simulink library "thc"  (R2021b)
settings: Solver=VariableStepAuto  StartTime=0.0  StopTime=10.0  RelTol=1e-3
undefined symbols (not defined in the file or in its folder): ATHC_APTCQA_X_C, ATHC_APTCQB_X_C, ATHC_dAy_X_C, ATHC_Qeq_X_kmh, ATHC_VbaseC_X_C, ATHC_VbaseC_Y_W, ATHC_VbaseD_X_C, ATHC_VbaseH_X_C, FALSE, KTHC_ACMaxMinT_sec, KTHC_aDeice_K, KTHC_AGSDefLv_K, KTHC_AGSLv1_K, KTHC_AGSLv2_K, KTHC_AGSLv3_K, KTHC_AGSLv4_K, KTHC_AGSLv5_K, KTHC_AirIntUpdateT_sec, KTHC_APTCOneZoneMax_W, KTHC_APTCPeriod_cnt, KTHC_APTCPWMEN_flg, KTHC_APTCQMaxC_W, KTHC_APTCQminC_W, KTHC_APTCQminD_W, KTHC_APTCQminRe1_W, KTHC_APTCQminRe_W, KTHC_APTCQoffT_cnt, KTHC_APTCQonT_cnt, KTHC_APTCRiLeMaxDff_W, KTHC_APTCRiLeMinDff_W, KTHC_BatInTempDef_C, KTHC_bDeice_K, KTHC_CompMaxDeice_rpm, KTHC_CompMinDeice_rpm, KTHC_CompSotxvOp_K, KTHC_CompSotxvOpLow_rpm, KTHC_CompSpdmax_rpm, KTHC_CompSpdmaxBC1_rpm, KTHC_CompSpdmaxBC_rpm, KTHC_CompSpdmid1_rpm, KTHC_CompSpdmid2_rpm, KTHC_CompSpdmid3_rpm, KTHC_CompSpdmid_rpm, KTHC_CompSpdmin_rpm, KTHC_DAPTCQ1_W, KTHC_DAPTCQ2_W, KTHC_DAPTCQ3_W, KTHC_DcChSetTemp_C, KTHC_DehumidityEN_flg, KTHC_DeiceCycTime_K, KTHC_DriveLevelWPTCBAH1_W, KTHC_DriveLevelWPTCBAH2_W, KTHC_DriveLevelWPTCBAH3_W, KTHC_DriveLevelWPTCBAH4_W, KTHC_DriveT1MinBAH_C, KTHC_DriveT2MaxBAH_C, KTHC_DriveT2MinBAH_C, KTHC_DriveT3MaxBAH_C, KTHC_DriveT3MinBAH_C, KTHC_DriveT4MaxBAH_C ... (+372)
libraries: simulink x140
(part 2 of 10)

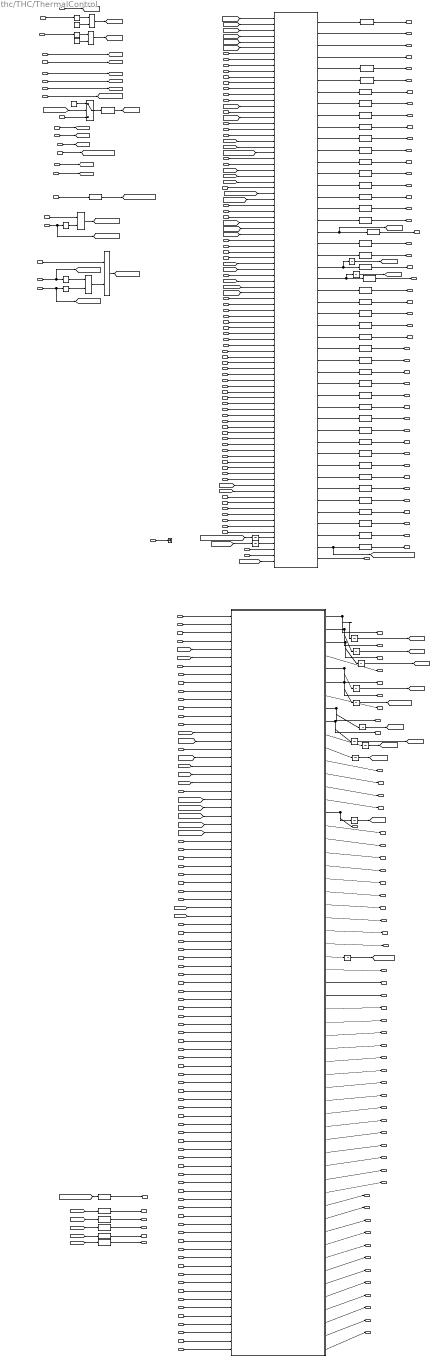
== system thc/THC/ThermalControl ==
  note: Ver Infomation
      | THCM Model V86test2A
      | ACHMI Model V27A
  VPMM_PwrSta_enum : Inport
  VTQD_ShiftGearPosn_enum : Inport  Port=2
  VSCP_AGSCloseSta_flg : Inport  Port=3
  VINP_VehSpeed_kph : Inport  Port=4
  VINP_HVBMTempMax_C : Inport  Port=5
  VINP_HVBMTempMin_C : Inport  Port=6
  VINP_OBCTemp_C : Inport  Port=7
  VINP_DCDCTemp_C : Inport  Port=8
  VINP_RrTMTemp_C : Inport  Port=9
  VINP_RrMCUTemp_C : Inport  Port=10
  VINP_FrTMTemp_C : Inport  Port=11
  VINP_FrMCUTemp_C : Inport  Port=12
  VINP_ChrgPlugSta_enum : Inport  Port=13
  VINP_FrLLCTemp_C : Inport  Port=14
  VINP_RrLLCTemp_C : Inport  Port=15
  VINP_HVBIsoImpedenceN_Mohm : Inport  Port=16
  VINP_HVBIsoImpedenceP_Mohm : Inport  Port=17
  VINP_HVBHVILErr_flg : Inport  Port=18
  VINP_HVBattSOC_pct : Inport  Port=19
  VINP_PTHighTact_C : Inport  Port=20
  VINP_COMP_StatorSpd_RPM : Inport  Port=21
  VINP_CompProEN_flg : Inport  Port=22
  VINP_PTLowP1_kPa : Inport  Port=23
  VINP_PTLowT1_C : Inport  Port=24
  VINP_PTLowP2_kPa : Inport  Port=25
  VINP_PTLowT2_C : Inport  Port=26
  VINP_PTHighP_kPa : Inport  Port=27
  VINP_Tamb_C : Inport  Port=28
  VINP_BatInTemp_C : Inport  Port=29
  VINP_BatOutTemp_C : Inport  Port=30
  VINP_MotorInTemp_C : Inport  Port=31
  VINP_MotorOutTemp_C : Inport  Port=32
  VINP_Tincar_C : Inport  Port=33
  VINP_SolarL_W : Inport  Port=34
  VINP_SolarR_W : Inport  Port=35
  VINP_Tevap_C : Inport  Port=36
  VINP_TFaceL_C : Inport  Port=37
  VINP_TFaceR_C : Inport  Port=38
  VINP_TFootL_C : Inport  Port=39
  VINP_TFootR_C : Inport  Port=40
  VINP_TFootRr_C : Inport  Port=41
  VINP_TFaceRr_C : Inport  Port=42
  VINP_EACProtectEnable_enum : Inport  Port=43
  Tamb_Err : Inport  Port=44
  SolarL_Err : Inport  Port=45
  SolarR_Err : Inport  Port=46
  Tevap_Err : Inport  Port=47
  T_Face_L_Err : Inport  Port=48
  T_Face_R_Err : Inport  Port=49
  T_Foot_L_Err : Inport  Port=50
  T_Foot_R_Err : Inport  Port=51
  T_Face_Rr_Err : Inport  Port=52
  T_Foot_Rr_Err : Inport  Port=53
  Tincar_Err : Inport  Port=54
  Bat_In_Temp_Err : Inport  Port=55
  Motor_In_Temp_Err : Inport  Port=56
  Motor_Out_Temp_Err : Inport  Port=57
  Fan_Err : Inport  Port=58
  AGS_Err : Inport  Port=59
  EWP3_Err : Inport  Port=60
  PT_High_P_Err : Inport  Port=61
  PT_High_Tact_Err : Inport  Port=62
  SOV1_Err : Inport  Port=63
  SOV2_Err : Inport  Port=64
  SOV3_Err : Inport  Port=65
  EXV1_Err : Inport  Port=66
  EXV2_Err : Inport  Port=67
  Comp_Err : Inport  Port=68
  Blower_Err : Inport  Port=69
  PT_Low_P1_Err : Inport  Port=70
  PT_Low_T1_Err : Inport  Port=71
  PT_Low_P2_Err : Inport  Port=72
  PT_Low_T2_Err : Inport  Port=73
  SOTXV_Err : Inport  Port=74
  VINP_FrntPTCRearLeActHeatPwr_W : Inport  Port=75
  VINP_FrntPTCRearRiActHeatPwr_W : Inport  Port=76
  VINP_FrntPTCRiActHeatPwr_W : Inport  Port=77
  VINP_ZFRTHCDrEVentActYSta_enum : Inport  Port=78
  VINP_ZFRTHCCLEVentActYSta_enum : Inport  Port=79
  VINP_ZFRTHCPsEVentActYSta_enum : Inport  Port=80
  VINP_ZFRTHCCREVentActYSta_enum : Inport  Port=81
  VINP_FGSAirIntSta_enum : Inport  Port=82
  VINP_FGSMotorInitSta_enum : Inport  Port=83
  VINP_OFFACMODE_enum : Inport  Port=84
  VINP_FCPFrEvtBtnACMaxReq_flg : Inport  Port=85
  VINP_FCPFrEvtBtnACReq_flg : Inport  Port=86
  VINP_FCPFrEvtBtnAutoReq_flg : Inport  Port=87
  VINP_FCPFrEvtBtnSyncReq_flg : Inport  Port=88
  VINP_sigAirIntenZon1Req_enum : Inport  Port=89
  VINP_sigRecircReq_flg : Inport  Port=90
  VINP_sigFaceReq_flg : Inport  Port=91
  VINP_sigFootReq_flg : Inport  Port=92
  VINP_sigFrostReq_flg : Inport  Port=93
  VINP_sigSetTempZon1Req_C : Inport  Port=94
  VINP_CANMsgValidIVI2_flg : Inport  Port=95
  VINP_sigSetTempZon2Req_C : Inport  Port=96
  VINP_SmartEcoModeSW_flg : Inport  Port=97
  VINP_HMIACBtnCmd_flg : Inport  Port=98
  VINP_HMIACAutoBtnCmd_flg : Inport  Port=99
  VINP_HMIACRecycleBtnCmd_flg : Inport  Port=100
  VINP_HMIACFrDefogBtnCmd_flg : Inport  Port=101
  VINP_HMIZ1SetTPCmd_flg : Inport  Port=102
  VINP_HMIZ1SetTMCmd_flg : Inport  Port=103
  VINP_HMIZ2SetTPCmd_flg : Inport  Port=104
  VINP_HMIZ2SetTMCmd_flg : Inport  Port=105
  VINP_HMIACWindDirPCmd_flg : Inport  Port=106
  VINP_HMIACWindDirMCmd_flg : Inport  Port=107
  VINP_HMIACAirIntPCmd_flg : Inport  Port=108
  VINP_HMIACAirIntDirMCmd_flg : Inport  Port=109
  VINP_IVIAirIntZ3Cmd_enum : Inport  Port=110
  VINP_IVIDrBlowerModeSta_enum : Inport  Port=111
  VINP_IVIPsBlowerModeSta_enum : Inport  Port=112
  VINP_IVIDrBlowerZSta_enum : Inport  Port=113
  VINP_IVICLBlowerZSta_enum : Inport  Port=114
  VINP_IVIPsBlowerZSta_enum : Inport  Port=115
  VINP_IVICRBlowerZSta_enum : Inport  Port=116
  VINP_IVIDrBlowerYSta_enum : Inport  Port=117
  VINP_IVICLBlowerYSta_enum : Inport  Port=118
  VINP_IVIPsBlowerYSta_enum : Inport  Port=119
  VINP_IVICRBlowerYSta_enum : Inport  Port=120
  VINP_IVIsigScreenReq_Sta : Inport  Port=121
  VINP_IVIFGSAirIntCmd_enum : Inport  Port=122
  VINP_IVIFGSChCmd_enum : Inport  Port=123
  VINP_IVIIONSWCmd_flg : Inport  Port=124
  VINP_IVIWPTCSWSta_flg : Inport  Port=125
  VINP_IVIZon1WindDirSWReqSta_flg : Inport  Port=126
  ECOSW : Inport  Port=127
  EEP_ACModeMem : Inport  Port=128
  EEP_Face : Inport  Port=129
  EEP_Foot : Inport  Port=130
  EEP_Frost : Inport  Port=131
  EEP_FaceM : Inport  Port=132
  EEP_FootM : Inport  Port=133
  EEP_CCUSyncSts : Inport  Port=134
  EEP_ACForceOFF : Inport  Port=135
  EEP_sigRecircSt : Inport  Port=136
  EEP_RecAutoFlg : Inport  Port=137
  EEP_AirIntenZone1iM : Inport  Port=138
  EEP_fdefog : Inport  Port=139
  EEP_sigSetTempZon1St : Inport  Port=140
  EEP_sigSetTempZon2StM : Inport  Port=141
  EEP_FDCTHCAirIntZ3Sta : Inport  Port=142
  VINP_FDCTHCPsEVentModeStaM_enum : Inport  Port=143
  VINP_FDCTHCDrEVentModeStaM_enum : Inport  Port=144
  VINP_FDCTHCDrEVentZStaM_enum : Inport  Port=145
  VINP_FDCTHCCLEVentZStaM_enum : Inport  Port=146
  VINP_FDCTHCPsEVentZStaM_enum : Inport  Port=147
  VINP_FDCTHCCREVentZStaM_enum : Inport  Port=148
  EEP_DrVentENM : Inport  Port=149
  VINP_FDCTHCDrEVentYStaM_enum : Inport  Port=150
  EEP_CLVentENM : Inport  Port=151
  VINP_FDCTHCCLEVentYStaM_enum : Inport  Port=152
  EEP_PsVentENM : Inport  Port=153
  VINP_FDCTHCPsEVentYStaM_enum : Inport  Port=154
  EEP_CRVentENM : Inport  Port=155
  VINP_FDCTHCCREVentYStaM_enum : Inport  Port=156
  FGSAirIntStaM : Inport  Port=157
  FGSChStaM : Inport  Port=158
  "IONSWStaM " : Inport  Port=159
  APTCFailDTC : Inport  Port=160
  VINP_RemoteACTemp_C : Inport  Port=161
  VINP_RemoteAutoReq_flg : Inport  Port=162
  AC1 : Subsystem
  Abs : Abs
  Abs1 : Abs
  Constant : Constant
  Constant1 : Constant
  Constant2 : Constant  Value=2
  Data Type Conversion{,1..47,50} (49 alike) : DataTypeConversion
  Data Type Conversion48 : DataTypeConversion  OutDataTypeStr=uint8
  Data Type Conversion49 : DataTypeConversion  OutDataTypeStr=uint16
  Logical Operator : Logic  Operator=OR  AllPortsSameDT=off  OutDataTypeStr=boolean
  Logical Operator1 : Logic  Operator=OR  AllPortsSameDT=off  OutDataTypeStr=boolean
  Logical Operator2 : Logic  AllPortsSameDT=off  OutDataTypeStr=boolean
  Logical Operator3 : Logic  Operator=NOT  AllPortsSameDT=off  OutDataTypeStr=boolean
  Logical Operator4 : Logic  Operator=NOT  AllPortsSameDT=off  OutDataTypeStr=boolean
  Logical Operator5 : Logic  Operator=NOT  AllPortsSameDT=off  OutDataTypeStr=boolean
  Max : MinMax  Function=max  Inputs=2
  Max1 : MinMax  Function=max  Inputs=2
  Switch : Switch  Criteria=u2 > Threshold
  THCM_Conctrl : Subsystem
  Terminator : Terminator
  Unit Delay{,1..14} (15 alike) : UnitDelay  SampleTime=-1  HasFrameUpgradeWarning=on
  VTHC_FDCompCmd_rpm : Outport
  VTHC_FDSOV1Cmd_flg : Outport  Port=2
  VTHC_FDSOV2Cmd_flg : Outport  Port=3
  VTHC_FDSOV3Cmd_flg : Outport  Port=4
  VTHC_FDEXV1Cmd_step : Outport  Port=5
  VTHC_FDEXV2Cmd_step : Outport  Port=6
  VTHC_FDSOTXVCmd_flg : Outport  Port=7
  VTHC_FDFWVCmd_flg : Outport  Port=8
  VTHC_FDTWVCmd_pct : Outport  Port=9
  VTHC_FDFrWPTCHeatPwrCmd_W : Outport  Port=10
  VTHC_CoolgFanActDuty_pct : Outport  Port=11
  VTHC_FDAGSCmd_enum : Outport  Port=12
  VTHC_FDEWP1Cmd_enum : Outport  Port=13
  VTHC_FDEWP2Cmd_enum : Outport  Port=14
  VTHC_FDEWP3Cmd_enum : Outport  Port=15
  VTHC_FDFrLeAPTCHeatPwrCmd_W : Outport  Port=16
  VTHC_FDFrRiAPTCHeatPwrCmd_W : Outport  Port=17
  VTHC_FDRrAPTCHeatPwrCmd_W : Outport  Port=18
  VTHC_FDBlowerCmd_pct : Outport  Port=19
  VTHC_BatteryMode_enum : Outport  Port=20
  VTHC_EDriveMode_enum : Outport  Port=21
  VTHC_CabinMode_enum : Outport  Port=22
  VTHC_CCUACLampSts_flg : Outport  Port=23
  VTHC_CCUAutoLampSts_flg : Outport  Port=24
  VTHC_CCUACMaxLampSts_flg : Outport  Port=25
  VTHC_CCUSyncLampSts_flg : Outport  Port=26
  VTHC_sigAirIntenZon1St_enum : Outport  Port=27
  VTHC_sigWindDirZon1St_enum : Outport  Port=28
  VTHC_sigRecircSt_flg : Outport  Port=29
  VTHC_sigSetTempZon1St_C : Outport  Port=30
  VTHC_sigSetTempZon2St_C : Outport  Port=31
  VTHC_sigClntTHvBattOut_C : Outport  Port=32
  VTHC_sigCbnSolarLeft_W : Outport  Port=33
  VTHC_sigClntTHvBattIn_C : Outport  Port=34
  VTHC_sigCbnSolarRight_W : Outport  Port=35
  VTHC_sigAmbAirT_C : Outport  Port=36
  VTHC_sigCbnAirT_C : Outport  Port=37
  VTHC_ACSubMode_enum : Outport  Port=38
  VTHC_FDRecyAutoCmd_enum : Outport  Port=39
  VTHC_CompP_K : Outport  Port=40
  VTHC_CompI_K : Outport  Port=41
  VTHC_CompU_K : Outport  Port=42
  VTHC_CompDeltaU_K : Outport  Port=43
  VTHC_Compe_K : Outport  Port=44
  VTHC_Blowere_K : Outport  Port=45
  VTHC_BlowerP_K : Outport  Port=46
  VTHC_BlowerU_K : Outport  Port=47
  VTHC_Vbase_pct : Outport  Port=48
  VTHC_BlowerI_K : Outport  Port=49
  VTHC_EXV2P_K : Outport  Port=50
  VTHC_EXV2I_K : Outport  Port=51
  VTHC_EXV2U_K : Outport  Port=52
  VTHC_EXV2e_K : Outport  Port=53
  VTHC_APTCP_K : Outport  Port=54
  VTHC_APTCI_K : Outport  Port=55
  VTHC_APTCU_K : Outport  Port=56
  VTHC_APTCe_K : Outport  Port=57
  VTHC_EXV1P_K : Outport  Port=58
  VTHC_EXV1I_K : Outport  Port=59
  VTHC_EXV1U_K : Outport  Port=60
  VTHC_EXV1e_K : Outport  Port=61
  VTHC_ACModeMem_enum : Outport  Port=62
  VTHC_Face_flg : Outport  Port=63
  VTHC_Foot_flg : Outport  Port=64
  VTHC_Frost_flg : Outport  Port=65
  VTHC_FaceM_flg : Outport  Port=66
  VTHC_FootM_flg : Outport  Port=67
  VTHC_CCUSyncSts_flg : Outport  Port=68
  VTHC_ACForceOFF_flg : Outport  Port=69
  VTHC_RecAutoFlg_flg : Outport  Port=70
  VTHC_AirIntenZone1M_enum : Outport  Port=71
  VTHC_fdefog_flg : Outport  Port=72
  VTHC_sigSetTempZon2StM_C : Outport  Port=73
  VTHC_sigDfrstSt_flg : Outport  Port=74
  VTHC_FDCTHCAirIntZ3Sta_enum : Outport  Port=75
  VTHC_FDCTHCDrEVentModeSta_enum : Outport  Port=76
  VTHC_FDCTHCPsEVentModeSta_enum : Outport  Port=77
  VTHC_FDCTHCDrEVentZSta_enum : Outport  Port=78
  VTHC_FDCTHCCLEVentZSta_enum : Outport  Port=79
  VTHC_FDCTHCPsEVentZSta_enum : Outport  Port=80
  VTHC_FDCTHCCREVentZSta_enum : Outport  Port=81
  VTHC_FDCTHCDrEVentYSta_enum : Outport  Port=82
  VTHC_FDCTHCDrVentENSta_flg : Outport  Port=83
  VTHC_FDCTHCCLEVentYSta_enum : Outport  Port=84
  VTHC_FDCTHCCLVentENSta_flg : Outport  Port=85
  VTHC_FDCTHCPsEVentYSta_enum : Outport  Port=86
  VTHC_FDCTHCPsVentENSta_flg : Outport  Port=87
  VTHC_FDCTHCCREVentYSta_enum : Outport  Port=88
  VTHC_FDCTHCCRVentENSta_flg : Outport  Port=89
  VTHC_FDCTHCMAPTCForceOFFSta_flg : Outport  Port=90
  VTHC_DrVentEN_flg : Outport  Port=91
  VTHC_CLVentEN_flg : Outport  Port=92
  VTHC_PsVentEN_flg : Outport  Port=93
  VTHC_CRVentEN_flg : Outport  Port=94
  VTHC_Z1TUP_flg : Outport  Port=95
  VTHC_Z1TDN_flg : Outport  Port=96
  VTHC_Z2TUP_flg : Outport  Port=97
  VTHC_Z2TDN_flg : Outport  Port=98
  VTHC_FDCFGSAirIntSta_enum : Outport  Port=99
  VTHC_FDCFGSChSta_enum : Outport  Port=100
  VTHC_FDCFGSAirIntCmd_enum : Outport  Port=101
  VTHC_FDCFGSFuncSta_flg : Outport  Port=102
  VTHC_FDCFGSChCmd_enum : Outport  Port=103
  VTHC_FDCFGSIONSWSta_flg : Outport  Port=104
  VTHC_FDCFGSIONCmd_flg : Outport  Port=105
  VTHC_FDCFGSLearnCmd_enum : Outport  Port=106
  VTHC_FDCTHCMPreWPTCHeatSta_enum : Outport  Port=107
  wires:
  AC1/9(VTHC_sigSetTempZon2St_C) -> Unit Delay9/1, VTHC_sigSetTempZon2St_C/1
  AC1/2(VTHC_CCUAutoLampSts_flg) -> Unit Delay2/1, VTHC_CCUAutoLampSts_flg/1
  AC1/6(VTHC_sigWindDirZon1St_enum) -> Unit Delay14/1, VTHC_sigWindDirZon1St_enum/1
  Unit Delay3/1 -> [ACMAX]
  AC1/4(VTHC_CCUSyncLampSts_flg) -> VTHC_CCUSyncLampSts_flg/1
  AC1/1(VTHC_CCUACLampSts_flg) -> Unit Delay1/1, VTHC_CCUACLampSts_flg/1
  AC1/5(VTHC_sigAirIntenZon1St_enum) -> Unit Delay4/1, VTHC_sigAirIntenZon1St_enum/1
  AC1/8(VTHC_sigSetTempZon1St_C) -> Unit Delay5/1, VTHC_sigSetTempZon1St_C/1
  THCM_Conctrl/19(FD_Blower_Cmd) -> Data Type Conversion/1, [FD_Blower_Cmd]
  Unit Delay5/1 -> [sigSetTempZon1St]
  AC1/7(VTHC_sigRecircSt_flg) -> VTHC_sigRecircSt_flg/1
  AC1/3(VTHC_CCUACMaxLampSts_flg) -> Unit Delay3/1, VTHC_CCUACMaxLampSts_flg/1
  VPMM_PwrSta_enum/1 -> [PwrSta]
  THCM_Conctrl/13(FD_EWP1_Cmd) -> Data Type Conversion3/1
  THCM_Conctrl/11(CoolgFanActDuty) -> Data Type Conversion1/1
  THCM_Conctrl/18(FD_RrAPTCHeatPwr_Cmd) -> Data Type Conversion8/1
  THCM_Conctrl/21(EDriveMode) -> Data Type Conversion22/1
  THCM_Conctrl/20(BatteryMode) -> Data Type Conversion21/1
  THCM_Conctrl/16(FD_FrLeAPTCHeatPwr_Cmd) -> Data Type Conversion6/1
  VINP_Tincar_C/1 -> [Tincar]
  THCM_Conctrl/9(FD_TWV_Cmd) -> Data Type Conversion19/1
  THCM_Conctrl/4(FD_SOV3_Cmd) -> VTHC_FDSOV3Cmd_flg/1
  VINP_SolarR_W/1 -> [SolarR]
  THCM_Conctrl/15(FD_EWP3_Cmd) -> Data Type Conversion5/1
  THCM_Conctrl/2(FD_SOV1_Cmd) -> VTHC_FDSOV1Cmd_flg/1
  Unit Delay2/1 -> [ACAUTO]
  THCM_Conctrl/7(FD_SOTXV_Cmd) -> Data Type Conversion46/1
  THCM_Conctrl/14(FD_EWP2_Cmd) -> Data Type Conversion4/1
  THCM_Conctrl/3(FD_SOV2_Cmd) -> VTHC_FDSOV2Cmd_flg/1
  THCM_Conctrl/6(FD_EXV2_Cmd) -> Data Type Conversion17/1
  VINP_Tamb_C/1 -> [Tamb]
  THCM_Conctrl/8(FD_FWV_Cmd) -> Data Type Conversion18/1
  VINP_BatInTemp_C/1 -> [BatInTemp]
  Unit Delay1/1 -> [AC]
  THCM_Conctrl/17(FD_FrRiAPTCHeatPwr_Cmd) -> Data Type Conversion7/1
  VINP_SolarL_W/1 -> [SolarL]
  THCM_Conctrl/12(FD_AGS_Cmd) -> Data Type Conversion2/1
  VINP_TFootL_C/1 -> [TFootL]
  Unit Delay4/1 -> [sigAirIntenZon1St]
  THCM_Conctrl/10(FD_FrWPTCHeatPwr_Cmd) -> Data Type Conversion20/1
  THCM_Conctrl/22(CabinMode) -> Unit Delay11/1, Data Type Conversion23/1
  [SolarL] -> Data Type Conversion41/1  "VTHC_sigCbnSolarLeft_W"
  [SolarR] -> Data Type Conversion43/1  "VTHC_sigCbnSolarRight_W"
  [BatInTemp] -> Data Type Conversion42/1  "VTHC_sigClntTHvBattIn_C"
  [Tamb] -> Data Type Conversion44/1  "VTHC_sigAmbAirT_C"
  [Tincar] -> Data Type Conversion45/1  "VTHC_sigCbnAirT_C"
  VINP_PTLowP2_kPa/1 -> Abs/1
  Abs/1 -> Max/1
  Constant/1 -> Max/2
  Constant1/1 -> Max1/2
  Abs1/1 -> Max1/1
  VINP_PTLowP1_kPa/1 -> Abs1/1
  VINP_TFootR_C/1 -> [TFootR]
  VINP_TFootRr_C/1 -> [TFootRr]
  VINP_CompProEN_flg/1 -> [VINP_CompProEN_flg]
  THCM_Conctrl/23(ACSubMode) -> Data Type Conversion28/1, Unit Delay/1
  THCM_Conctrl/24(VTHC_CompP_K) -> Data Type Conversion29/1
  THCM_Conctrl/25(VTHC_CompI_K) -> Data Type Conversion35/1
  THCM_Conctrl/26(VTHC_CompU_K) -> Data Type Conversion36/1
  THCM_Conctrl/27(VTHC_CompDeltaU_K) -> Data Type Conversion34/1
  THCM_Conctrl/28(VTHC_Compe_K) -> Data Type Conversion33/1
  THCM_Conctrl/29(VTHC_Blowere_K) -> Data Type Conversion32/1
  THCM_Conctrl/30(VTHC_BlowerP_K) -> Data Type Conversion31/1
  THCM_Conctrl/31(VTHC_BlowerU_K) -> Data Type Conversion30/1
  THCM_Conctrl/32(VTHC_Vbase_pct) -> Data Type Conversion37/1
  THCM_Conctrl/33(VTHC_BlowerI_K) -> Data Type Conversion38/1
  THCM_Conctrl/34(VTHC_EXV2P_K) -> Data Type Conversion24/1
  THCM_Conctrl/35(VTHC_EXV2I_K) -> Data Type Conversion25/1
  THCM_Conctrl/36(VTHC_EXV2U_K) -> Data Type Conversion26/1
  THCM_Conctrl/37(VTHC_EXV2e_K) -> Data Type Conversion27/1
  THCM_Conctrl/39(VTHC_APTCI_K) -> Data Type Conversion16/1
  THCM_Conctrl/40(VTHC_APTCU_K) -> Data Type Conversion15/1
  THCM_Conctrl/41(VTHC_APTCe_K) -> Data Type Conversion14/1
  THCM_Conctrl/42(VTHC_EXV1P_K) -> Data Type Conversion11/1
  THCM_Conctrl/43(VTHC_EXV1I_K) -> Data Type Conversion12/1
  THCM_Conctrl/44(VTHC_EXV1U_K) -> Data Type Conversion13/1
  THCM_Conctrl/45(VTHC_EXV1e_K) -> Data Type Conversion9/1
  THCM_Conctrl/5(FD_EXV1_Cmd) -> Data Type Conversion10/1
  Data Type Conversion1/1 -> VTHC_CoolgFanActDuty_pct/1  "CoolgFanActDuty"
  Data Type Conversion2/1 -> VTHC_FDAGSCmd_enum/1  "FD_AGS_Cmd"
  Data Type Conversion3/1 -> VTHC_FDEWP1Cmd_enum/1  "FD_EWP1_Cmd"
  Data Type Conversion4/1 -> VTHC_FDEWP2Cmd_enum/1  "FD_EWP2_Cmd"
  Data Type Conversion5/1 -> VTHC_FDEWP3Cmd_enum/1  "FD_EWP3_Cmd"
  Data Type Conversion6/1 -> VTHC_FDFrLeAPTCHeatPwrCmd_W/1  "FD_FrLeAPTCHeatPwr_Cmd"
  Data Type Conversion8/1 -> VTHC_FDRrAPTCHeatPwrCmd_W/1  "FD_RrAPTCHeatPwr_Cmd"
  Data Type Conversion7/1 -> VTHC_FDFrRiAPTCHeatPwrCmd_W/1  "FD_FrRiAPTCHeatPwr_Cmd"
  Data Type Conversion9/1 -> VTHC_EXV1e_K/1  "VTHC_EXV1e_K"
  Data Type Conversion10/1 -> VTHC_FDEXV1Cmd_step/1  "FD_EXV1_Cmd"
  Data Type Conversion11/1 -> VTHC_EXV1P_K/1  "VTHC_EXV1P_K"
  Data Type Conversion12/1 -> VTHC_EXV1I_K/1  "VTHC_EXV1I_K"
  Data Type Conversion13/1 -> VTHC_EXV1U_K/1  "VTHC_EXV1U_K"
  Data Type Conversion14/1 -> VTHC_APTCe_K/1  "VTHC_APTCe_K"
  Data Type Conversion15/1 -> VTHC_APTCU_K/1  "VTHC_APTCU_K"
  Data Type Conversion16/1 -> VTHC_APTCI_K/1  "VTHC_APTCI_K"
  THCM_Conctrl/38(VTHC_APTCP_K) -> Data Type Conversion39/1
  Data Type Conversion17/1 -> VTHC_FDEXV2Cmd_step/1  "FD_EXV2_Cmd"
  Data Type Conversion18/1 -> VTHC_FDFWVCmd_flg/1  "FD_FWV_Cmd"
  Data Type Conversion19/1 -> VTHC_FDTWVCmd_pct/1  "FD_TWV_Cmd"
  Data Type Conversion20/1 -> VTHC_FDFrWPTCHeatPwrCmd_W/1  "FD_FrWPTCHeatPwr_Cmd"
  Data Type Conversion21/1 -> VTHC_BatteryMode_enum/1  "BatteryMode"
  Data Type Conversion22/1 -> VTHC_EDriveMode_enum/1  "EDriveMode"
  Data Type Conversion23/1 -> VTHC_CabinMode_enum/1  "CabinMode"
  Data Type Conversion24/1 -> VTHC_EXV2P_K/1  "VTHC_EXV2P_K"
  Data Type Conversion25/1 -> VTHC_EXV2I_K/1  "VTHC_EXV2I_K"
  Data Type Conversion26/1 -> VTHC_EXV2U_K/1  "VTHC_EXV2U_K"
  Data Type Conversion27/1 -> VTHC_EXV2e_K/1  "VTHC_EXV2e_K"
  Data Type Conversion28/1 -> VTHC_ACSubMode_enum/1  "ACSubMode"
  Data Type Conversion29/1 -> VTHC_CompP_K/1  "VTHC_CompP_K"
  Data Type Conversion30/1 -> VTHC_BlowerU_K/1  "VTHC_BlowerU_K"
  Data Type Conversion31/1 -> VTHC_BlowerP_K/1  "VTHC_BlowerP_K"
  Data Type Conversion32/1 -> VTHC_Blowere_K/1  "VTHC_Blowere_K"
  Data Type Conversion33/1 -> VTHC_Compe_K/1  "VTHC_Compe_K"
  Data Type Conversion34/1 -> VTHC_CompDeltaU_K/1  "VTHC_CompDeltaU_K"
  Data Type Conversion35/1 -> VTHC_CompI_K/1  "VTHC_CompI_K"
  Data Type Conversion36/1 -> VTHC_CompU_K/1  "VTHC_CompU_K"
  Data Type Conversion37/1 -> VTHC_Vbase_pct/1  "VTHC_Vbase_pct"
  Data Type Conversion38/1 -> VTHC_BlowerI_K/1  "VTHC_BlowerI_K"
  Data Type Conversion39/1 -> VTHC_APTCP_K/1  "VTHC_APTCP_K"
  Data Type Conversion40/1 -> VTHC_sigClntTHvBattOut_C/1  "VINP_BatOutTemp_C"
  Data Type Conversion41/1 -> VTHC_sigCbnSolarLeft_W/1  "SolarL"
  Data Type Conversion42/1 -> VTHC_sigClntTHvBattIn_C/1  "BatInTemp"
  Data Type Conversion43/1 -> VTHC_sigCbnSolarRight_W/1  "SolarR"
  Data Type Conversion44/1 -> VTHC_sigAmbAirT_C/1  "Tamb"
  Data Type Conversion45/1 -> VTHC_sigCbnAirT_C/1  "Tincar"
  AC1/10(WaterFillReq) -> Unit Delay7/1
  AC1/16(Frost) -> Unit Delay8/1, VTHC_Frost_flg/1
  Unit Delay8/1 -> [DfrstReq]
  Unit Delay7/1 -> [WaterFillReq]
  Unit Delay9/1 -> [sigSetTempZon2St]
  Data Type Conversion/1 -> VTHC_FDBlowerCmd_pct/1
  Data Type Conversion46/1 -> VTHC_FDSOTXVCmd_flg/1
  VINP_BatOutTemp_C/1 -> [VINP_BatOutTemp_C]
  [VINP_BatOutTemp_C] -> Data Type Conversion40/1
  AC1/11(PET) -> Unit Delay10/1
  Unit Delay10/1 -> [PET]
  THCM_Conctrl/1(FD_Comp_Cmd) -> Data Type Conversion47/1
  Data Type Conversion47/1 -> VTHC_FDCompCmd_rpm/1  "VTHC_FDCompCmd_rpm"
  Unit Delay11/1 -> [CabinMode]
  AC1/12(FD_RecyAuto_Cmd) -> VTHC_FDRecyAutoCmd_enum/1
  [VINP_CompProEN_flg] -> Switch/2
  Switch/1 -> Data Type Conversion48/1
  Constant2/1 -> Switch/1
  VINP_EACProtectEnable_enum/1 -> Switch/3
  Max1/1 -> [PTLowP1]
  Max/1 -> [PTLowP2]
  [PwrSta] -> THCM_Conctrl/1(PwrSta)
  [AC] -> THCM_Conctrl/2(AC)
  [ACMAX] -> THCM_Conctrl/3(ACMax)
  [ACAUTO] -> THCM_Conctrl/4(ACAuto)
  [sigSetTempZon1St] -> THCM_Conctrl/5(sigSetTempZon1St)
  [sigAirIntenZon1St] -> THCM_Conctrl/6(sigAirIntenZon1St)
  VINP_VehSpeed_kph/1 -> THCM_Conctrl/7(VehSpeed)
  VINP_HVBMTempMax_C/1 -> THCM_Conctrl/8(HVBMTempMax)
  VINP_HVBMTempMin_C/1 -> THCM_Conctrl/9(HVBMTempMin)
  [PTLowP1] -> THCM_Conctrl/16(PT_ Low_P1)
  VINP_OBCTemp_C/1 -> THCM_Conctrl/10(OBCTemp)
  VINP_DCDCTemp_C/1 -> THCM_Conctrl/11(DCDCTemp)
  [PTLowP2] -> THCM_Conctrl/18(PT_Low_P2)
  VINP_RrTMTemp_C/1 -> THCM_Conctrl/12(Rr_TMTemp)
  VINP_RrMCUTemp_C/1 -> THCM_Conctrl/13(Rr_MCUTemp)
  VINP_FrTMTemp_C/1 -> THCM_Conctrl/14(Fr_TMTemp)
  VINP_FrMCUTemp_C/1 -> THCM_Conctrl/15(Fr_MCUTemp)
  [VINP_BatOutTemp_C] -> THCM_Conctrl/24(Bat_Out_Temp)
  [Tamb] -> THCM_Conctrl/22(Tamb)
  VINP_PTLowT1_C/1 -> THCM_Conctrl/17(PT_ Low_T1)
  [BatInTemp] -> THCM_Conctrl/23(Bat_In_Temp)
  VINP_PTLowT2_C/1 -> THCM_Conctrl/19(PT_ Low_T2)
  VINP_PTHighP_kPa/1 -> THCM_Conctrl/20(PT_High_P)
  VINP_PTHighTact_C/1 -> THCM_Conctrl/21(PT_High_Tact)
  [Tincar] -> THCM_Conctrl/27(Tincar)
  [SolarL] -> THCM_Conctrl/28(SolarL)
  [VINP_CompProEN_flg] -> THCM_Conctrl/32(CompProEN)
  [SolarR] -> THCM_Conctrl/29(SolarR)
  VINP_MotorInTemp_C/1 -> THCM_Conctrl/25(Motor_In_Temp)
  VINP_MotorOutTemp_C/1 -> THCM_Conctrl/26(Motor_Out_Temp)
  VINP_Tevap_C/1 -> THCM_Conctrl/30(Tevap)
  VINP_COMP_StatorSpd_RPM/1 -> Data Type Conversion49/1
  [DfrstReq] -> THCM_Conctrl/36(DfrstReq)
  VSCP_AGSCloseSta_flg/1 -> THCM_Conctrl/33(VSCP_AGSCloseSta_flg)
  [WaterFillReq] -> THCM_Conctrl/37(WaterFillReq)
  VTQD_ShiftGearPosn_enum/1 -> THCM_Conctrl/34(ShiftGearPosn)
  [sigSetTempZon2St] -> THCM_Conctrl/38(sigSetTempZon2St)
  VINP_ChrgPlugSta_enum/1 -> THCM_Conctrl/35(ChrgPlugSta)
  [TFootR] -> THCM_Conctrl/44(T_Foot_R)
  VINP_FrLLCTemp_C/1 -> THCM_Conctrl/39(Fr_LLCTemp)
  [TFootL] -> THCM_Conctrl/43(T_Foot_L)
  VINP_RrLLCTemp_C/1 -> THCM_Conctrl/40(Rr_LLCTemp)
  VINP_TFaceL_C/1 -> THCM_Conctrl/41(T_Face_L)
  [PET] -> THCM_Conctrl/47(PET)
  [TFootRr] -> THCM_Conctrl/46(T_Foot_Rr)
  [EACProtectEnable] -> THCM_Conctrl/48(EACProtectEnable)
  VINP_TFaceR_C/1 -> THCM_Conctrl/42(T_Face_R)
  VINP_TFaceRr_C/1 -> THCM_Conctrl/45(T_Face_Rr)
  Tamb_Err/1 -> THCM_Conctrl/49(Tamb_Err)
  SolarL_Err/1 -> THCM_Conctrl/50(SolarL_Err)
  SolarR_Err/1 -> THCM_Conctrl/51(SolarR_Err)
  Tevap_Err/1 -> THCM_Conctrl/52(Tevap_Err)
  T_Face_L_Err/1 -> THCM_Conctrl/53(T_Face_L_Err)
  T_Face_R_Err/1 -> THCM_Conctrl/54(T_Face_R_Err)
  T_Foot_L_Err/1 -> THCM_Conctrl/55(T_Foot_L_Err)
  T_Foot_R_Err/1 -> THCM_Conctrl/56(T_Foot_R_Err)
  T_Face_Rr_Err/1 -> THCM_Conctrl/57(T_Face_Rr_Err)
  T_Foot_Rr_Err/1 -> THCM_Conctrl/58(T_Foot_Rr_Err)
  Tincar_Err/1 -> THCM_Conctrl/59(Tincar_Err)
  Bat_In_Temp_Err/1 -> THCM_Conctrl/60(Bat_In_Temp_Err)
  Motor_In_Temp_Err/1 -> THCM_Conctrl/61(Motor_In_Temp_Err)
  Motor_Out_Temp_Err/1 -> THCM_Conctrl/62(Motor_Out_Temp_Err)
  Fan_Err/1 -> THCM_Conctrl/63(Fan_Err)
  AGS_Err/1 -> THCM_Conctrl/64(AGS_Err)
  EWP3_Err/1 -> THCM_Conctrl/65(EWP3_Err)
  PT_High_P_Err/1 -> THCM_Conctrl/66(PT_High_P_Err)
  PT_High_Tact_Err/1 -> THCM_Conctrl/67(PT_High_Tact_Err)
  SOV1_Err/1 -> THCM_Conctrl/68(SOV1_Err)
  SOV2_Err/1 -> THCM_Conctrl/69(SOV2_Err)
  SOV3_Err/1 -> THCM_Conctrl/70(SOV3_Err)
  EXV1_Err/1 -> THCM_Conctrl/71(EXV1_Err)
  EXV2_Err/1 -> THCM_Conctrl/72(EXV2_Err)
  Comp_Err/1 -> THCM_Conctrl/73(Comp_Err)
  Blower_Err/1 -> THCM_Conctrl/74(Blower_Err)
  PT_Low_P1_Err/1 -> THCM_Conctrl/75(PT_Low_P1_Err)
  PT_Low_T1_Err/1 -> THCM_Conctrl/76(PT_Low_T1_Err)
  PT_Low_P2_Err/1 -> THCM_Conctrl/77(PT_Low_P2_Err)
  PT_Low_T2_Err/1 -> THCM_Conctrl/78(PT_Low_T2_Err)
  SOTXV_Err/1 -> THCM_Conctrl/79(SOTXV_Err)
  VINP_FCPFrEvtBtnACMaxReq_flg/1 -> AC1/1(VINP_FCPFrEvtBtnACMaxReq_flg)
  VINP_FCPFrEvtBtnACReq_flg/1 -> AC1/2(VINP_FCPFrEvtBtnACReq_flg)
  [Tamb] -> AC1/5(VINP_Tamb_C)
  VINP_FCPFrEvtBtnAutoReq_flg/1 -> AC1/3(VINP_FCPFrEvtBtnAutoReq_flg)
  [Tincar] -> AC1/6(VINP_Tincar_C)
  VINP_FCPFrEvtBtnSyncReq_flg/1 -> AC1/4(VINP_FCPFrEvtBtnSyncReq_flg)
  VINP_sigAirIntenZon1Req_enum/1 -> AC1/7(VINP_sigAirIntenZon1Req_enum)
  VINP_sigRecircReq_flg/1 -> AC1/8(VINP_sigRecircReq_flg)
  VINP_sigFaceReq_flg/1 -> AC1/9(VINP_sigFaceReq_flg)
  VINP_sigFootReq_flg/1 -> AC1/10(VINP_sigFootReq_flg)
  VINP_sigFrostReq_flg/1 -> AC1/11(VINP_sigFrostReq_flg)
  VINP_sigSetTempZon1Req_C/1 -> AC1/12(VINP_sigSetTempZon1Req_C)
  [FD_Blower_Cmd] -> AC1/15(VTHC_FDBlowerCmd_pct)
  VINP_CANMsgValidIVI2_flg/1 -> AC1/13(VINP_CANMsgValidIVI2_flg)
  [PwrSta] -> AC1/16(PwrSta)
  VINP_sigSetTempZon2Req_C/1 -> AC1/14(VINP_sigSetTempZon2Req_C)
  [CabinMode] -> AC1/18(CabinMode)
  [TFootL] -> AC1/19(T_Foot_L)
  VINP_OFFACMODE_enum/1 -> AC1/17(OFF_AC_MODE)
  [TFootR] -> AC1/20(T_Foot_R)
  [TFootRr] -> AC1/21(T_Foot_Rr)
  EEP_ACModeMem/1 -> AC1/22(EEP_ACModeMem)
  AC1/13(ACModeMem) -> VTHC_ACModeMem_enum/1
  AC1/14(Face) -> VTHC_Face_flg/1
  AC1/15(Foot) -> VTHC_Foot_flg/1
  AC1/17(FaceM) -> VTHC_FaceM_flg/1
  AC1/18(FootM) -> VTHC_FootM_flg/1
  AC1/19(CCUSyncSts) -> VTHC_CCUSyncSts_flg/1
  AC1/20(ACForceOFF) -> VTHC_ACForceOFF_flg/1
  AC1/22(AirIntenZone1M) -> VTHC_AirIntenZone1M_enum/1
  AC1/23(fdefog) -> VTHC_fdefog_flg/1
  EEP_CCUSyncSts/1 -> AC1/28(EEP_CCUSyncSts)
  EEP_ACForceOFF/1 -> AC1/29(EEP_ACForceOFF)
  EEP_sigRecircSt/1 -> AC1/30(EEP_sigRecircSt)
  EEP_RecAutoFlg/1 -> AC1/31(EEP_RecAutoFlg)
  EEP_AirIntenZone1iM/1 -> AC1/32(EEP_AirIntenZone1M)
  EEP_fdefog/1 -> AC1/33(EEP_fdefog)
  EEP_sigSetTempZon1St/1 -> AC1/34(EEP_sigSetTempZon1Req)
  EEP_sigSetTempZon2StM/1 -> AC1/35(EEP_sigSetTempZon2StM)
  AC1/21(RecAutoFlg) -> VTHC_RecAutoFlg_flg/1
  AC1/24(VTHC_sigSetTempZon2StM_C) -> VTHC_sigSetTempZon2StM_C/1
  ECOSW/1 -> THCM_Conctrl/80(ECOSW)
  VINP_RemoteACTemp_C/1 -> [RemoteACTemp]
  [RemoteACTemp] -> THCM_Conctrl/81(RemoteACTemp)
  VINP_RemoteAutoReq_flg/1 -> [RemoteAutoReq]
  [RemoteAutoReq] -> THCM_Conctrl/82(RemoteAutoReq)
  [RemoteAutoReq] -> AC1/36(VINP_RemoteAutoReq_flg)
  Unit Delay/1 -> [ACSubMode]
  [ACSubMode] -> AC1/37(ACSubMode)
  Data Type Conversion48/1 -> [EACProtectEnable]
  Data Type Conversion49/1 -> [VINP_COMP_StatorSpd_RPM]
  [VINP_COMP_StatorSpd_RPM] -> THCM_Conctrl/31(CompFB)
  EEP_FootM/1 -> [EEP_FootM], Logical Operator3/1
  EEP_FaceM/1 -> Logical Operator/1
  Logical Operator/1 -> [EEP_FaceM]
  [EEP_FaceM] -> AC1/26(EEP_FaceM)
  [EEP_FootM] -> AC1/27(EEP_FootM)
  Logical Operator5/1 -> Logical Operator2/2
  EEP_Foot/1 -> [EEP_Foot], Logical Operator4/1
  EEP_Frost/1 -> [EEP_Frost], Logical Operator5/1
  Logical Operator2/1 -> Logical Operator1/2
  EEP_Face/1 -> Logical Operator1/1
  Logical Operator1/1 -> [EEP_Face]
  [EEP_Face] -> AC1/23(EEP_Face)
  [EEP_Frost] -> AC1/25(EEP_Frost)
  [EEP_Foot] -> AC1/24(EEP_Foot)
  Logical Operator3/1 -> Logical Operator/2
  Logical Operator4/1 -> Logical Operator2/1
  VINP_SmartEcoModeSW_flg/1 -> THCM_Conctrl/83(VINP_SmartEcoModeSW_flg)
  VINP_HVBIsoImpedenceN_Mohm/1 -> THCM_Conctrl/84(VINP_HVBIsoImpedenceN_Mohm)
  VINP_HVBIsoImpedenceP_Mohm/1 -> THCM_Conctrl/85(VINP_HVBIsoImpedenceP_Mohm)
  VINP_HVBHVILErr_flg/1 -> THCM_Conctrl/86(VINP_HVBHVILErr_flg)
  VINP_FrntPTCRearLeActHeatPwr_W/1 -> THCM_Conctrl/87(VINP_FrntPTCRearLeActHeatPwr_W)
  VINP_FrntPTCRearRiActHeatPwr_W/1 -> THCM_Conctrl/88(VINP_FrntPTCRearRiActHeatPwr_W)
  VINP_FrntPTCRiActHeatPwr_W/1 -> THCM_Conctrl/89(VINP_FrntPTCRiActHeatPwr_W)
  Unit Delay6/1 -> THCM_Conctrl/91(RrAPTCEN)
  AC1/25(VTHC_sigDfrstSt_flg) -> VTHC_sigDfrstSt_flg/1
  AC1/26(VTHC_FDCTHCAirIntZ3Sta_enum) -> VTHC_FDCTHCAirIntZ3Sta_enum/1
  AC1/27(RrAPTCEN) -> Unit Delay12/1
  Unit Delay12/1 -> [RrAPTCEN]
  [RrAPTCEN] -> Unit Delay6/1
  AC1/28(VTHC_FDCTHCDrEVentModeSta_enum) -> VTHC_FDCTHCDrEVentModeSta_enum/1  "VTHC_FDCTHCDrEVentModeSta_enum"
  AC1/29(VTHC_FDCTHCPsEVentModeSta_enum) -> VTHC_FDCTHCPsEVentModeSta_enum/1  "VTHC_FDCTHCPsEVentModeSta_enum"
  AC1/30(VTHC_FDCTHCDrEVentZSta_enum) -> VTHC_FDCTHCDrEVentZSta_enum/1  "VTHC_FDCTHCDrEVentZSta_enum"
  AC1/31(VTHC_FDCTHCCLEVentZSta_enum) -> VTHC_FDCTHCCLEVentZSta_enum/1  "VTHC_FDCTHCCLEVentZSta_enum"
  AC1/32(VTHC_FDCTHCPsEVentZSta_enum) -> VTHC_FDCTHCPsEVentZSta_enum/1  "VTHC_FDCTHCPsEVentZSta_enum"
  AC1/33(VTHC_FDCTHCCREVentZSta_enum) -> VTHC_FDCTHCCREVentZSta_enum/1  "VTHC_FDCTHCCREVentZSta_enum"
  AC1/34(VTHC_FDCTHCDrEVentYSta_enum) -> VTHC_FDCTHCDrEVentYSta_enum/1  "VTHC_FDCTHCDrEVentYSta_enum"
  AC1/35(VTHC_FDCTHCDrVentENSta_flg) -> VTHC_FDCTHCDrVentENSta_flg/1  "VTHC_FDCTHCDrVentENSta_flg"
  AC1/36(VTHC_FDCTHCCLEVentYSta_enum) -> VTHC_FDCTHCCLEVentYSta_enum/1  "VTHC_FDCTHCCLEVentYSta_enum"
  AC1/37(VTHC_FDCTHCCLVentENSta_flg) -> VTHC_FDCTHCCLVentENSta_flg/1  "VTHC_FDCTHCCLVentENSta_flg"
  AC1/38(VTHC_FDCTHCPsEVentYSta_enum) -> VTHC_FDCTHCPsEVentYSta_enum/1  "VTHC_FDCTHCPsEVentYSta_enum"
  AC1/39(VTHC_FDCTHCPsVentENSta_flg) -> VTHC_FDCTHCPsVentENSta_flg/1  "VTHC_FDCTHCPsVentENSta_flg"
  AC1/40(VTHC_FDCTHCCREVentYSta_enum) -> VTHC_FDCTHCCREVentYSta_enum/1  "VTHC_FDCTHCCREVentYSta_enum"
  AC1/41(VTHC_FDCTHCCRVentENSta_flg) -> VTHC_FDCTHCCRVentENSta_flg/1  "VTHC_FDCTHCCRVentENSta_flg"
  VINP_HMIACBtnCmd_flg/1 -> AC1/38(VINP_HMIACBtnCmd_flg)
  VINP_HMIACAutoBtnCmd_flg/1 -> AC1/39(VINP_HMIACAutoBtnCmd_flg)
  VINP_HMIACRecycleBtnCmd_flg/1 -> AC1/40(VINP_HMIACRecycleBtnCmd_flg)
  VINP_HMIACFrDefogBtnCmd_flg/1 -> AC1/41(VINP_HMIACFrDefogBtnCmd_flg)
  VINP_HMIZ1SetTPCmd_flg/1 -> AC1/42(VINP_HMIZ1SetTPCmd_flg)
  VINP_HMIZ1SetTMCmd_flg/1 -> AC1/43(VINP_HMIZ1SetTMCmd_flg)
  VINP_HMIZ2SetTPCmd_flg/1 -> AC1/44(VINP_HMIZ2SetTPCmd_flg)
  VINP_HMIZ2SetTMCmd_flg/1 -> AC1/45(VINP_HMIZ2SetTMCmd_flg)
  VINP_HMIACWindDirPCmd_flg/1 -> AC1/46(VINP_HMIACWindDirPCmd_flg)
  VINP_HMIACWindDirMCmd_flg/1 -> AC1/47(VINP_HMIACWindDirMCmd_flg)
  VINP_HMIACAirIntPCmd_flg/1 -> AC1/48(VINP_HMIACAirIntPCmd_flg)
  VINP_HMIACAirIntDirMCmd_flg/1 -> AC1/49(VINP_HMIACAirIntDirMCmd_flg)
  VINP_IVIAirIntZ3Cmd_enum/1 -> AC1/50(VINP_IVIAirIntZ3Cmd_enum)
  EEP_FDCTHCAirIntZ3Sta/1 -> AC1/51(EEP_FDCTHCAirIntZ3Sta)
  VINP_IVIDrBlowerModeSta_enum/1 -> AC1/52(VINP_IVIDrBlowerModeSta_enum)
  VINP_IVIPsBlowerModeSta_enum/1 -> AC1/53(VINP_IVIPsBlowerModeSta_enum)
  VINP_IVIDrBlowerZSta_enum/1 -> AC1/54(VINP_IVIDrBlowerZSta_enum)
  VINP_IVICLBlowerZSta_enum/1 -> AC1/55(VINP_IVICLBlowerZSta_enum)
  VINP_IVIPsBlowerZSta_enum/1 -> AC1/56(VINP_IVIPsBlowerZSta_enum)
  VINP_IVICRBlowerZSta_enum/1 -> AC1/57(VINP_IVICRBlowerZSta_enum)
  VINP_IVIDrBlowerYSta_enum/1 -> AC1/58(VINP_IVIDrBlowerYSta_enum)
  VINP_IVICLBlowerYSta_enum/1 -> AC1/59(VINP_IVICLBlowerYSta_enum)
  VINP_IVIPsBlowerYSta_enum/1 -> AC1/60(VINP_IVIPsBlowerYSta_enum)
  VINP_IVICRBlowerYSta_enum/1 -> AC1/61(VINP_IVICRBlowerYSta_enum)
  VINP_ZFRTHCDrEVentActYSta_enum/1 -> AC1/62(VINP_ZFRTHCDrEVentActYSta_enum)
  VINP_ZFRTHCCLEVentActYSta_enum/1 -> AC1/63(VINP_ZFRTHCCLEVentActYSta_enum)
  VINP_ZFRTHCPsEVentActYSta_enum/1 -> AC1/64(VINP_ZFRTHCPsEVentActYSta_enum)
  VINP_ZFRTHCCREVentActYSta_enum/1 -> AC1/65(VINP_ZFRTHCCREVentActYSta_enum)
  VINP_FDCTHCDrEVentModeStaM_enum/1 -> AC1/66(VINP_FDCTHCDrEVentModeStaM_enum)
  VINP_FDCTHCPsEVentModeStaM_enum/1 -> AC1/67(VINP_FDCTHCPsEVentModeStaM_enum)
  VINP_FDCTHCDrEVentZStaM_enum/1 -> AC1/68(VINP_FDCTHCDrEVentZStaM_enum)
  VINP_FDCTHCCLEVentZStaM_enum/1 -> AC1/69(VINP_FDCTHCCLEVentZStaM_enum)
  VINP_FDCTHCPsEVentZStaM_enum/1 -> AC1/70(VINP_FDCTHCPsEVentZStaM_enum)
  VINP_FDCTHCCREVentZStaM_enum/1 -> AC1/71(VINP_FDCTHCCREVentZStaM_enum)
  EEP_DrVentENM/1 -> AC1/72(EEP_DrVentENM)
  VINP_FDCTHCDrEVentYStaM_enum/1 -> AC1/73(VINP_FDCTHCDrEVentYStaM_enum)
  EEP_CLVentENM/1 -> AC1/74(EEP_CLVentENM)
  VINP_FDCTHCCLEVentYStaM_enum/1 -> AC1/75(VINP_FDCTHCCLEVentYStaM_enum)
  EEP_PsVentENM/1 -> AC1/76(EEP_PsVentENM)
  VINP_FDCTHCPsEVentYStaM_enum/1 -> AC1/77(VINP_FDCTHCPsEVentYStaM_enum)
  EEP_CRVentENM/1 -> AC1/78(EEP_CRVentENM)
  VINP_FDCTHCCREVentYStaM_enum/1 -> AC1/79(VINP_FDCTHCCREVentYStaM_enum)
  VINP_IVIsigScreenReq_Sta/1 -> AC1/80(VINP_IVIsigScreenReq_Sta)
  Data Type Conversion50/1 -> VTHC_FDCTHCMAPTCForceOFFSta_flg/1  "VTHC_FDCTHCMAPTCForceOFFSta_flg"
  THCM_Conctrl/46(VTHC_FDCTHCMAPTCForceOFFSta_flg) -> [VTHC_FDCTHCMAPTCForceOFFSta_flg], Data Type Conversion50/1
  APTCFailDTC/1 -> Terminator/1
  Unit Delay13/1 -> THCM_Conctrl/90(APTCFailDTC)
  [VTHC_FDCTHCMAPTCForceOFFSta_flg] -> Unit Delay13/1
  AC1/43(VTHC_CLVentEN_flg) -> VTHC_CLVentEN_flg/1  "VTHC_CLVentEN_flg"
  AC1/42(VTHC_DrVentEN_flg) -> VTHC_DrVentEN_flg/1  "VTHC_DrVentEN_flg"
  AC1/45(VTHC_CRVentEN_flg) -> VTHC_CRVentEN_flg/1  "VTHC_CRVentEN_flg"
  AC1/44(VTHC_PsVentEN_flg) -> VTHC_PsVentEN_flg/1  "VTHC_PsVentEN_flg"
  VINP_IVIFGSAirIntCmd_enum/1 -> AC1/81(VINP_IVIFGSAirIntCmd_enum)
  FGSAirIntStaM/1 -> AC1/82(FGSAirIntStaM)
  VINP_IVIFGSChCmd_enum/1 -> AC1/83(VINP_IVIFGSChCmd_enum)
  FGSChStaM/1 -> AC1/84(FGSChStaM)
  VINP_IVIIONSWCmd_flg/1 -> AC1/85(VINP_IVIIONSWCmd_flg)
  "IONSWStaM "/1 -> AC1/86("IONSWStaM ")
  VINP_FGSMotorInitSta_enum/1 -> AC1/87(VINP_FGSMotorInitSta_enum)
  VINP_FGSAirIntSta_enum/1 -> AC1/88(VINP_FGSAirIntSta_enum)
  AC1/46(VTHC_Z1TUP_flg) -> VTHC_Z1TUP_flg/1
  AC1/47(VTHC_Z1TDN_flg) -> VTHC_Z1TDN_flg/1
  AC1/48(VTHC_Z2TUP_flg) -> VTHC_Z2TUP_flg/1
  AC1/49(VTHC_Z2TDN_flg) -> VTHC_Z2TDN_flg/1
  AC1/50(VTHC_FDCFGSAirIntSta_enum) -> VTHC_FDCFGSAirIntSta_enum/1
  AC1/51(VTHC_FDCFGSChSta_enum) -> VTHC_FDCFGSChSta_enum/1
  AC1/52(VTHC_FDCFGSAirIntCmd_enum) -> VTHC_FDCFGSAirIntCmd_enum/1
  AC1/53(VTHC_FDCFGSFuncSta_flg) -> VTHC_FDCFGSFuncSta_flg/1
  AC1/54(VTHC_FDCFGSChCmd_enum) -> VTHC_FDCFGSChCmd_enum/1
  AC1/55(VTHC_FDCFGSIONSWSta_flg) -> VTHC_FDCFGSIONSWSta_flg/1
  AC1/56(VTHC_FDCFGSIONCmd_flg) -> VTHC_FDCFGSIONCmd_flg/1
  AC1/57(VTHC_FDCFGSLearnCmd_enum) -> VTHC_FDCFGSLearnCmd_enum/1
  Unit Delay14/1 -> [sigWindDirZon1St]
  [sigWindDirZon1St] -> THCM_Conctrl/94(sigWindDirZon1St)
  VINP_HVBattSOC_pct/1 -> THCM_Conctrl/92(VINP_HVBattSOC_pct)
  VINP_IVIWPTCSWSta_flg/1 -> THCM_Conctrl/93(VINP_IVIWPTCSWSta_flg)
  THCM_Conctrl/47(VTHC_FDCTHCMPreWPTCHeatSta_enum) -> VTHC_FDCTHCMPreWPTCHeatSta_enum/1
  VINP_IVIZon1WindDirSWReqSta_flg/1 -> AC1/89(VINP_IVIZon1WindDirSWReqSta_flg)
